simulink model "Controlador_Lazo_abierto"  (R2019b)
settings: Solver=VariableStepAuto  StartTime=0.0  StopTime=10.0  RelTol=1e-3
values from neighbouring files (symbols this model uses):
  alfa = 2    [Lazo_abierto.m]    (also in lazo_abierto.m; lazo_cerrado.m; main.m)
  K_c = omega_n^2 * K_g    (= 147)    [Lazo_abierto.m]    (also in lazo_abierto.m; lazo_cerrado.m = 0.0058319; main.m)
  K_g = 3    [Lazo_abierto.m]    (also in lazo_abierto.m; lazo_cerrado.m; main.m)
  omega_n = 7    [Lazo_abierto.m]    (also in lazo_abierto.m; lazo_cerrado.m; main.m)
  Per_A = 0.1    [Lazo_abierto.m]    (also in lazo_abierto.m; main.m)
  Per_freq = 5    [Lazo_abierto.m]    (also in lazo_abierto.m; main.m)
  Tau = sqrt(1/(Limite_u * K_c))    [Lazo_abierto.m]    (also in lazo_abierto.m; main.m)
  xi = 0.5    [Lazo_abierto.m]    (also in lazo_abierto.m; lazo_cerrado.m; main.m)
settings Model: Creator=toman  LastModifiedBy=toman

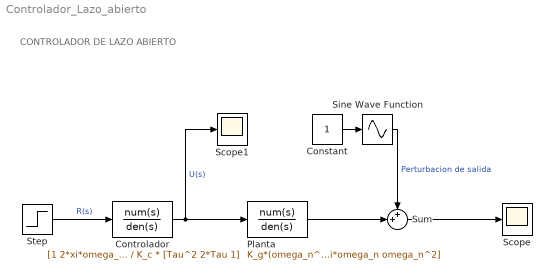
== system Controlador_Lazo_abierto ==
  note: CONTROLADOR DE LAZO ABIERTO
  Constant : Constant
  "Controlador " : TransferFcn  Numerator=[1 2*xi*omega_n omega_n^2]  Denominator=K_c * [Tau^2 2*Tau 1]
  "Planta " : TransferFcn  Numerator=K_g*(omega_n^2)*[-1*alfa 1]  Denominator=[1 2*xi*omega_n omega_n^2]
  Scope : Scope
  Scope1 : Scope
  Sine Wave Function : Sin  TimeSource=Use external signal  Amplitude=Per_A  Frequency=Per_freq  SampleTime=0
  Step : Step  SampleTime=0
  Sum : Sum  Inputs=++|
  wires:
  Step/1 -> "Controlador "/1  "R(s)"
  "Planta "/1 -> Sum/2
  Sine Wave Function/1 -> Sum/1  "Perturbacion de salida"
  Sum/1 -> Scope/1
  "Controlador "/1 -> "Planta "/1, Scope1/1  "U(s)"
  Constant/1 -> Sine Wave Function/1
